simulink library "DRC_SimulinkLibrary"  (R2021a)
settings: Solver=VariableStepAuto  StartTime=0.0  StopTime=10.0  RelTol=1e-3
undefined symbols (not defined in the file or in its folder): DiscIntNeverNeededParam, Ts, WSE
libraries: $bdroot x2, aerolibconvert2 x1
settings Model: Creator=Sebastiaan  LastModifiedBy=sebastiaanmuld

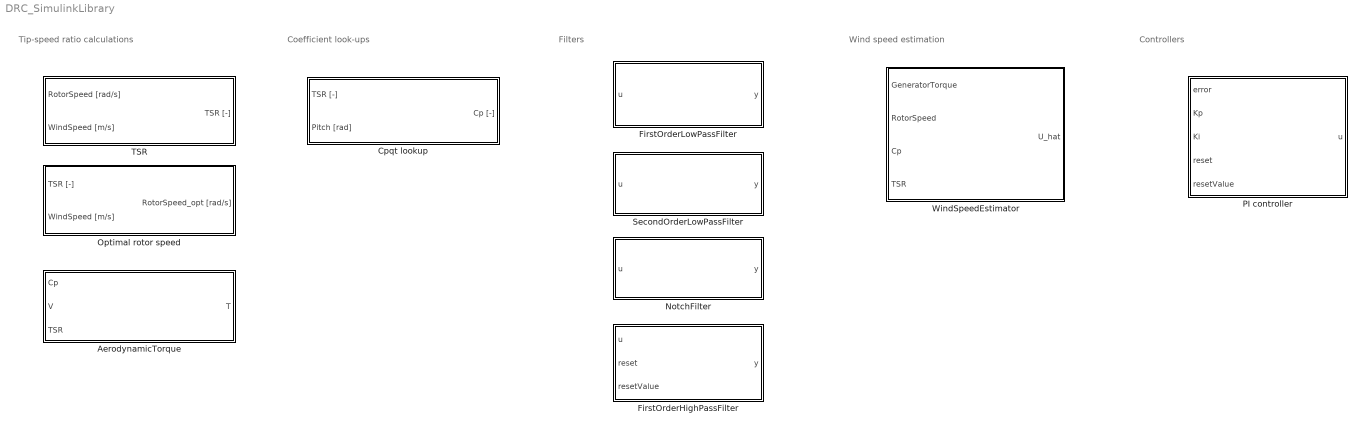
== system DRC_SimulinkLibrary ==
  note: Filters
  note: Coefficient look-ups
  note: Tip-speed ratio calculations
  note: Controllers
  note: Wind speed estimation
  AerodynamicTorque : Subsystem  mask{T=[]}
      mask prompts: T "Turbine properties struct"
  Cpqt lookup : Subsystem  mask(Coefficient look-up){CpqtGrid=[], TSRVector=[], PitchVector=[]}
      mask prompts: CpqtGrid "Cp/Cq/Ct grid [-]"; TSRVector "TSR vector [-]"; PitchVector "Pitch vector [-]"
      mask help: Coefficient look-up table for power coefficient (Cp), torque coefficient (Cq), and thrust coefficient (Ct). The TSR and Pitch data should be a 1-dimensional vector of sizes p and q, respectively. The provided coefficient matrix should be of size p x q.
  FirstOrderHighPassFilter : Subsystem  mask(First order high-pass filter){wc=-1, Ts=-1}
      mask prompts: wc "Cut-off frequency [rad/s]"; Ts "Sampling time [s]"
      mask help:
      | Discrete time notch filter (IIR), given in continuous time by:
      | G =  s / (s + wc)
      | with wc the cut-off frequency, and s the Laplace operator.
      |
      | Discretized using the bilinear transform (Tustin's method). The sampling time should be explicitly specified.
  FirstOrderLowPassFilter : Subsystem  mask(First order low-pass filter){wn=-1, Ts=-1}
      mask prompts: wn "Cut-off frequency [rad/s]"; Ts "Sampling time [s]"
      mask help:
      | Discrete time first order low-pass filter (IIR), given in continuous time by:
      | G = wc / ( s + wc)
      | with wc the cut-off frequency, and s the Laplace operator.
      |
      | Discretized using the bilinear transform (Tustin's method). The sampling time should be explicitly specified.
  NotchFilter : Subsystem  mask{wn=-1, betaNum=-1, betaDen=-1, Ts=-1}
      mask prompts: wn "Cut-off frequency [rad/s]"; betaNum "Beta numerator [-]"; betaDen "Beta denominator [-]"; Ts "Sampling time [s]"
      mask help:
      | Discrete time notch filter (IIR), given in continuous time by:
      | G =  ( s^2 + 2*wc*betaNum*s + wc^2 ) / ( s^2 + 2*wc*betaDen*s + wc^2 )
      | with wc the cut-off frequency, betaNum and betaDen being the damping coefficients, and s the Laplace operator. The ratio and magnitude of the ratio determines the width and depth of the notch.
      |
      | Discretized using the bilinear transform (Tustin's method). The sampling time should be explicitly specified.
  Optimal rotor speed : Subsystem  mask{RotorRadius=-1}
      mask prompts: RotorRadius "Rotor radius [m]"
  PI controller : Subsystem  mask{minSatValue=-inf, maxSatValue=inf, Ts=Ts}
      mask prompts: minSatValue "Minimum saturation"; maxSatValue "Maximum saturation"; Ts "Sampling time [s]"
  SecondOrderLowPassFilter : Subsystem  mask(Second order low-pass filter){wn=-1, damp=-1, Ts=-1}
      mask prompts: wn "Cut-off frequency [rad/s]"; damp "Damping coefficient [-]"; Ts "Sampling time [s]"
      mask help:
      | Discrete time second order low-pass filter (IIR), given in continuous time by:
      | G = wc^2 / ( s^2 + 2*wc*zeta*s + wc^2)
      | with wc the cut-off frequency, zeta the damping coefficient, and s the Laplace operator.
      |
      | Discretized using the bilinear transform (Tustin's method). The sampling time should be explicitly specified.
  TSR : Subsystem  mask(Tip-speed ratio){RotorRadius=-1}
      mask prompts: RotorRadius "Rotor radius [m]"
      mask help: Calculates the tip-speed ratio based on rotor speed [rad/s] and wind speed [m/s] signals.
  WindSpeedEstimator : Subsystem  mask{omega_r_0=0, T=[], Kp=WSE.KpWSE.Kp, Ki=WSE.Ki}
      mask prompts: omega_r_0 "Rotor speed initial value"; T "Turbine properties struct"; Kp "Proportional gain"; Ki "Integral gain"

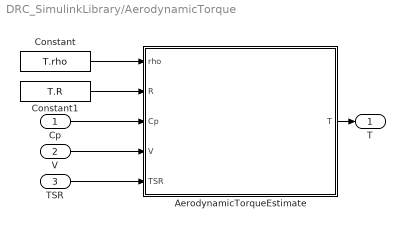
== system DRC_SimulinkLibrary/AerodynamicTorque ==
  Cp : Inport
  V : Inport  Port=2
  TSR : Inport  Port=3
  AerodynamicTorqueEstimate : MATLAB Function  TreatAsAtomicUnit=on
  Constant : Constant  Value=T.rho
  Constant1 : Constant  Value=T.R
  T : Outport
  wires:
  Constant/1 -> AerodynamicTorqueEstimate/1(rho)
  V/1 -> AerodynamicTorqueEstimate/4(V)
  AerodynamicTorqueEstimate/1(T) -> T/1
  Cp/1 -> AerodynamicTorqueEstimate/3(Cp)
  TSR/1 -> AerodynamicTorqueEstimate/5(TSR)
  Constant1/1 -> AerodynamicTorqueEstimate/2(R)

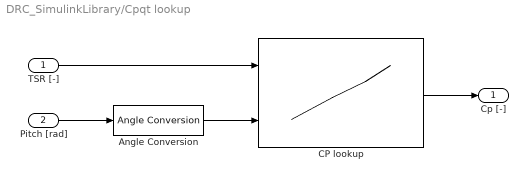
== system DRC_SimulinkLibrary/Cpqt lookup ==
  TSR [-] : Inport
  Pitch [rad] : Inport  Port=2
  Angle Conversion : aerolibconvert2/Angle Conversion  IU=rad  OU=deg
  CP lookup : Lookup_n-D  BreakpointsForDimension1=TSRVector  BreakpointsForDimension2=PitchVector  Table=CpqtGrid  InternalRulePriority=Speed  RndMeth=Simplest  InputSameDT=on
      settings: InputPortMap=u0,u1
  Cp [-] : Outport
  wires:
  Pitch [rad]/1 -> Angle Conversion/1
  Angle Conversion/1 -> CP lookup/2
  TSR [-]/1 -> CP lookup/1
  CP lookup/1 -> Cp [-]/1

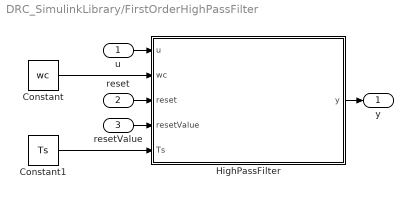
== system DRC_SimulinkLibrary/FirstOrderHighPassFilter ==
  u : Inport
  reset : Inport  Port=2
  resetValue : Inport  Port=3
  Constant : Constant  Value=wc
  Constant1 : Constant  Value=Ts
  HighPassFilter : MATLAB Function  TreatAsAtomicUnit=on
  y : Outport
  wires:
  HighPassFilter/1(y) -> y/1
  reset/1 -> HighPassFilter/3(reset)
  Constant/1 -> HighPassFilter/2(wc)
  Constant1/1 -> HighPassFilter/5(Ts)
  u/1 -> HighPassFilter/1(u)
  resetValue/1 -> HighPassFilter/4(resetValue)

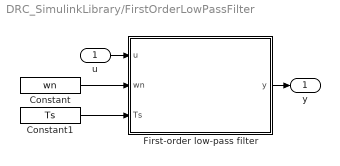
== system DRC_SimulinkLibrary/FirstOrderLowPassFilter ==
  u : Inport
  Constant : Constant  Value=wn
  Constant1 : Constant  Value=Ts
  First-order low-pass filter : MATLAB Function  TreatAsAtomicUnit=on
  y : Outport
  wires:
  Constant/1 -> First-order low-pass filter/2(wn)
  Constant1/1 -> First-order low-pass filter/3(Ts)
  First-order low-pass filter/1(y) -> y/1
  u/1 -> First-order low-pass filter/1(u)

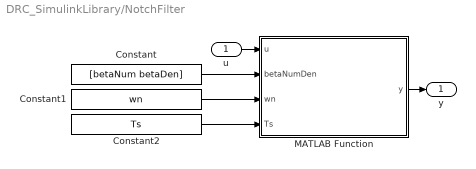
== system DRC_SimulinkLibrary/NotchFilter ==
  u : Inport
  Constant : Constant  Value=[betaNum betaDen]
  Constant1 : Constant  Value=wn
  Constant2 : Constant  Value=Ts
  MATLAB Function : MATLAB Function  TreatAsAtomicUnit=on
  y : Outport
  wires:
  Constant1/1 -> MATLAB Function/3(wn)
  MATLAB Function/1(y) -> y/1
  Constant2/1 -> MATLAB Function/4(Ts)
  Constant/1 -> MATLAB Function/2(betaNumDen)
  u/1 -> MATLAB Function/1(u)

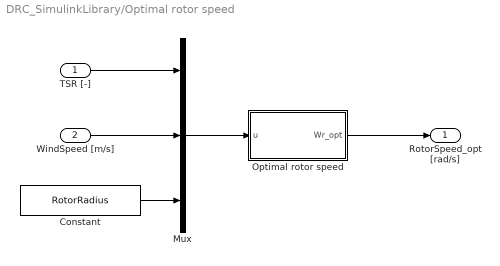
== system DRC_SimulinkLibrary/Optimal rotor speed ==
  TSR [-] : Inport
  WindSpeed [m/s] : Inport  Port=2
  Constant : Constant  Value=RotorRadius
  Mux : Mux  Inputs=3
  Optimal rotor speed : MATLAB Function  TreatAsAtomicUnit=on
  RotorSpeed_opt [rad/s] : Outport
  wires:
  Optimal rotor speed/1(Wr_opt) -> RotorSpeed_opt [rad/s]/1
  WindSpeed [m/s]/1 -> Mux/2
  Mux/1 -> Optimal rotor speed/1(u)
  Constant/1 -> Mux/3
  TSR [-]/1 -> Mux/1

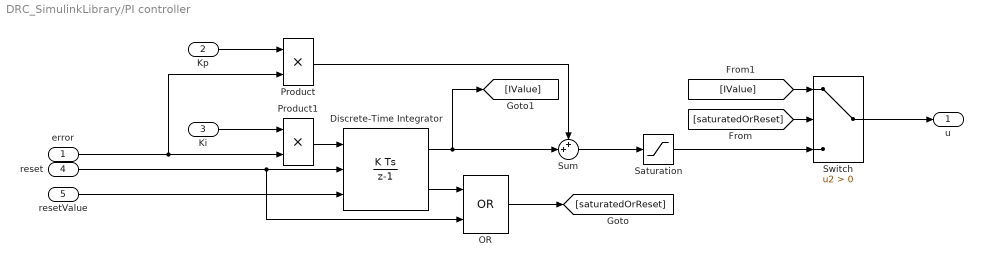
== system DRC_SimulinkLibrary/PI controller ==
  error : Inport
  Kp : Inport  Port=2
  Ki : Inport  Port=3
  reset : Inport  Port=4
  resetValue : Inport  Port=5
  Discrete-Time Integrator : DiscreteIntegrator  ExternalReset=level  InitialConditionSource=external  SampleTime=Ts  LimitOutput=on  UpperSaturationLimit=maxSatValue  LowerSaturationLimit=minSatValue  ShowSaturationPort=on  ICPrevOutput=DiscIntNeverNeededParam  ICPrevScaledInput=DiscIntNeverNeededParam
  OR : Logic  Operator=OR  AllPortsSameDT=off  OutDataTypeStr=boolean
  Product : Product
  Product1 : Product
  Saturation : Saturate  UpperLimit=maxSatValue  LowerLimit=minSatValue
  Sum : Sum  Inputs=++|
  Switch : Switch  Criteria=u2 > Threshold
  u : Outport
  wires:
  Product/1 -> Sum/1
  resetValue/1 -> Discrete-Time Integrator/3
  reset/1 -> OR/2, Discrete-Time Integrator/2
  Kp/1 -> Product/1
  Switch/1 -> u/1
  Discrete-Time Integrator/2 -> OR/1
  Discrete-Time Integrator/1 -> [IValue], Sum/2
  error/1 -> Product1/2, Product/2
  Product1/1 -> Discrete-Time Integrator/1
  Ki/1 -> Product1/1
  Sum/1 -> Saturation/1
  [saturatedOrReset] -> Switch/2
  [IValue] -> Switch/1
  Saturation/1 -> Switch/3
  OR/1 -> [saturatedOrReset]

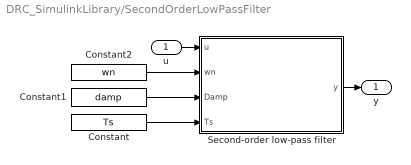
== system DRC_SimulinkLibrary/SecondOrderLowPassFilter ==
  u : Inport
  Constant : Constant  Value=Ts
  Constant1 : Constant  Value=damp
  Constant2 : Constant  Value=wn
  Second-order low-pass filter : MATLAB Function  TreatAsAtomicUnit=on
  y : Outport
  wires:
  u/1 -> Second-order low-pass filter/1(u)
  Constant2/1 -> Second-order low-pass filter/2(wn)
  Second-order low-pass filter/1(y) -> y/1
  Constant1/1 -> Second-order low-pass filter/3(Damp)
  Constant/1 -> Second-order low-pass filter/4(Ts)

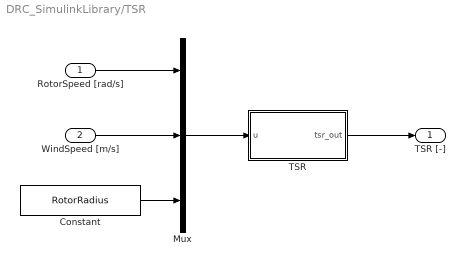
== system DRC_SimulinkLibrary/TSR ==
  RotorSpeed [rad/s] : Inport
  WindSpeed [m/s] : Inport  Port=2
  Constant : Constant  Value=RotorRadius
  Mux : Mux  Inputs=3
  TSR : MATLAB Function  TreatAsAtomicUnit=on
  TSR [-] : Outport
  wires:
  Constant/1 -> Mux/3
  Mux/1 -> TSR/1(u)
  WindSpeed [m/s]/1 -> Mux/2
  RotorSpeed [rad/s]/1 -> Mux/1
  TSR/1(tsr_out) -> TSR [-]/1

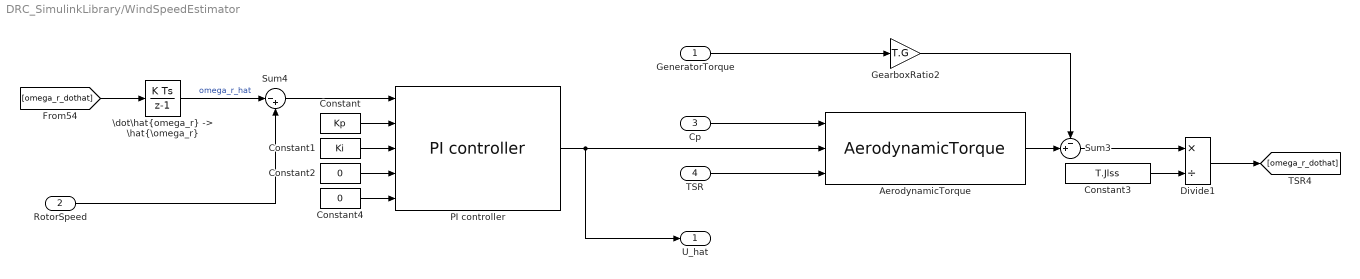
== system DRC_SimulinkLibrary/WindSpeedEstimator ==
  GeneratorTorque : Inport
  RotorSpeed : Inport  Port=2
  Cp : Inport  Port=3
  TSR : Inport  Port=4
  AerodynamicTorque : $bdroot/AerodynamicTorque  T=T
  Constant : Constant  Value=Kp
  Constant1 : Constant  Value=Ki
  Constant2 : Constant  Value=0
  Constant3 : Constant  Value=T.Jlss
  Constant4 : Constant  Value=0
  Divide1 : Product  Inputs=*/
  GearboxRatio2 : Gain  Gain=T.G
  PI controller : $bdroot/PI controller  maxSatValue=inf  minSatValue=-inf  Ts=-1
  Sum3 : Sum  Inputs=-+|
  Sum4 : Sum  Inputs=|-+
  "\\dot\\hat{omega_r} -> \\hat{\\omega_r}" : DiscreteIntegrator  InitialCondition=omega_r_0  SampleTime=-1  ICPrevOutput=DiscIntNeverNeededParam  ICPrevScaledInput=DiscIntNeverNeededParam
  U_hat : Outport
  wires:
  PI controller/1 -> AerodynamicTorque/2, U_hat/1
  Divide1/1 -> [omega_r_dothat]
  AerodynamicTorque/1 -> Sum3/2
  "\\dot\\hat{omega_r} -> \\hat{\\omega_r}"/1 -> Sum4/1  "omega_r_hat"
  GearboxRatio2/1 -> Sum3/1
  Constant3/1 -> Divide1/2
  Sum3/1 -> Divide1/1
  [omega_r_dothat] -> "\\dot\\hat{omega_r} -> \\hat{\\omega_r}"/1
  GeneratorTorque/1 -> GearboxRatio2/1
  RotorSpeed/1 -> Sum4/2
  Cp/1 -> AerodynamicTorque/1
  TSR/1 -> AerodynamicTorque/3
  Sum4/1 -> PI controller/1
  Constant/1 -> PI controller/2
  Constant1/1 -> PI controller/3
  Constant2/1 -> PI controller/4
  Constant4/1 -> PI controller/5

== matlab function DRC_SimulinkLibrary/Optimal rotor speed/Optimal rotor speed ==
  data: u input size=[1 3]; Wr_opt output
function Wr_opt = fcn(u)
    Wr_opt = tsr(u(1), u(2), u(3), 'WR');
end

== matlab function DRC_SimulinkLibrary/TSR/TSR ==
  data: u input size=[1 3]; tsr_out output
function tsr_out = fcn(u)
    tsr_out = tsr(u(1), u(2), u(3));
end

== matlab function DRC_SimulinkLibrary/AerodynamicTorque/AerodynamicTorqueEstimate ==
  data: rho input; R input; Cp input; T output; V input; TSR input
function T = aerodynamictorque(rho, R, Cp, V, TSR)

T = aerodynamictorque(rho, R, Cp, V, TSR);

== matlab function DRC_SimulinkLibrary/FirstOrderHighPassFilter/HighPassFilter ==
  data: u input; y output; wc input; reset input; resetValue input; Ts input
function y = fcn(u, wc, reset, resetValue, Ts)

    persistent u_prev1 y_prev1
    K = 2.0/Ts; % Constant gain
    
    if isempty(u_prev1) || reset
        u_prev1 = resetValue; % Initialize persistent input signal variable
        y_prev1 = resetValue; % Initialize persistent output signal variable
        
        y = resetValue;
    else
        y = K/(wc + K)*u - K/(wc + K)*u_prev1 - (wc - K)/(wc + K)*y_prev1;
        
        u_prev1 = u;
        y_prev1 = y;
    end

end

== matlab function DRC_SimulinkLibrary/SecondOrderLowPassFilter/Second-order low-pass filter ==
  data: u input; wn input; Damp input; y output; Ts input
function y = SecLPF(u, wn, Damp, Ts)

persistent y_prev1 y_prev2 u_prev1 u_prev2

if isempty(u_prev1)
    y_prev1 = u;
    y_prev2 = u;
    u_prev1 = u;
    u_prev2 = u;
end

y = 1/(4+4*Ts*Damp*wn+Ts^2*wn^2) * ( (8-2*Ts^2*wn^2)*y_prev1 + ...
    (-4+4*Ts*Damp*wn-Ts^2*wn^2)*y_prev2 + (Ts^2*wn^2)*u ...
    + (2*Ts^2*wn^2)*u_prev1 + (Ts^2*wn^2)*u_prev2 );

u_prev2   = u_prev1;
u_prev1   = u;
y_prev2  = y_prev1;
y_prev1  = y;

== matlab function DRC_SimulinkLibrary/FirstOrderLowPassFilter/First-order low-pass filter ==
  data: u input; wn input; y output; Ts input
function y = FirstLPF(u, wn, Ts)

persistent y_prev1 u_prev1

if isempty(u_prev1)
    y_prev1 = u;
    u_prev1 = u;
end

y = (Ts*wn*u + Ts*wn*u_prev1 - (Ts*wn-2.0)*y_prev1)/(Ts*wn+2.0);

u_prev1   = u;
y_prev1  = y;

== matlab function DRC_SimulinkLibrary/NotchFilter/MATLAB Function ==
  data: u input; betaNumDen input; wn input; y output; Ts input
function y = NotchFilter(u, betaNumDen, wn, Ts)

persistent u_prev1 u_prev2 y_prev1 y_prev2
if isempty(u_prev1)
    u_prev1 = u;
    u_prev2 = u;
    y_prev1 = u;
    y_prev2 = u;
end

if any([betaNumDen(1) betaNumDen(2) wn] == 0)
    y = u;
else
    % Prepare filter elements from current input
    K = 2/Ts;
    Part1 = (K^2 + 2*wn*betaNumDen(1) * K + wn^2) / (K^2 + 2*wn*betaNumDen(2) * K + wn^2);
    Part2 = (2 * wn^2 - 2 * K^2)  / (K^2 + 2*wn*betaNumDen(2) * K + wn^2);
    Part3 = (K^2 - 2*wn*betaNumDen(1) * K + wn^2) / (K^2 + 2*wn*betaNumDen(2) * K + wn^2);
    Part4 = (2 * wn^2 - 2 * K^2)  / (K^2 + 2*wn*betaNumDen(2) * K + wn^2);
    Part5 = (K^2 - 2*wn*betaNumDen(2)* K + wn^2)/ (K^2 + 2*wn*betaNumDen(2) * K + wn^2);
    
    % Compute filter output
    y = Part1*u + Part2*u_prev1 + Part3*u_prev2 - Part4*y_prev1 - Part5*y_prev2;
    
    % Save signals for next time step
    u_prev2 = u_prev1;
    u_prev1 = u;
    
    y_prev2 = y_prev1;
    y_prev1 = y;
end
